simulink model "lv_demo7"  (Simulink 7.1)
settings: Solver=ode45  StartTime=0.0  StopTime=100  RelTol=1e-3
values from neighbouring files (symbols this model uses):
  C1 = 0.44    [lv_demofile.m]    (also in lv_demofile1.m; lv_demofile2.m; lv_demofile4.m; lv_demofile5.m)
  C2 = 0.0167    [lv_demofile.m]    (also in lv_demofile1.m; lv_demofile2.m; lv_demofile4.m; lv_demofile5.m)
  C3 = 0.3    [lv_demofile.m]    (also in lv_demofile1.m; lv_demofile2.m; lv_demofile4.m; lv_demofile5.m)
  C4 = 0.00184    [lv_demofile.m]    (also in lv_demofile1.m; lv_demofile2.m; lv_demofile4.m; lv_demofile5.m)
  Jem = 90    [lv_cankaofile.m]    (also in lv_demofile.m = 97.5; lv_demofile1.m = 97.5; lv_demofile2.m = 97.5; lv_demofile3.m = 97.5)
  Jwt = 9e7    (= 90000000)    [lv_cankaofile.m]    (also in lv_demofile.m = 3275300; lv_demofile1.m = 3275300; lv_demofile2.m = 3275300; lv_demofile3.m = 3275300)
  K = 83    [lv_cankaofile.m]    (also in lv_demofile.m; lv_demofile1.m = 75.76; lv_demofile2.m; lv_demofile3.m = 75.76)
  R = 40    [lv_cankaofile.m]    (also in lv_demofile.m = 38.5; lv_demofile1.m = 38.75; lv_demofile2.m = 38.5; lv_demofile3.m = 38.5)
  ro_air = 1.225    [lv_cankaofile.m]    (also in lv_demofile.m = 1.2236; lv_demofile1.m; lv_demofile2.m = 1.2236; lv_demofile3.m)
libraries: wt_blockset_v3 x2, simulink x1
settings Model: Creator=lv  LastModifiedBy=lv

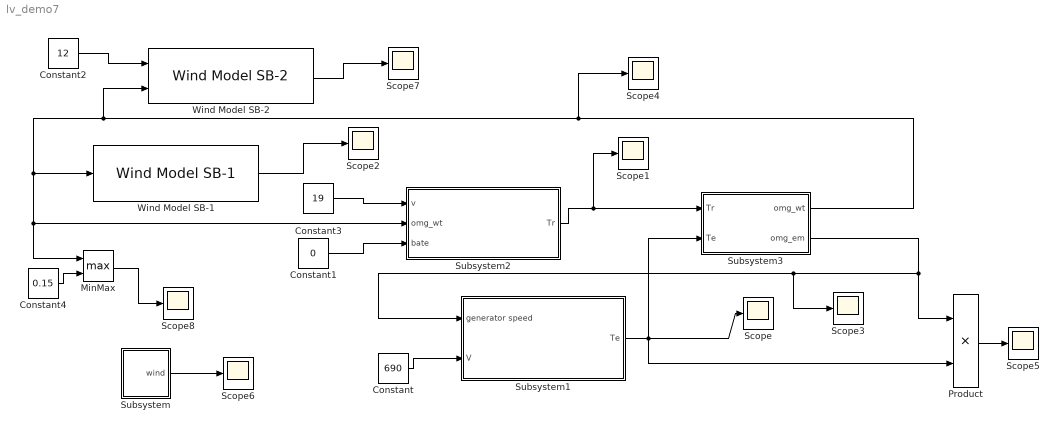
== system lv_demo7 ==
  Constant : Constant  Value=690  OutDataType=sfix(16)  OutScaling=2^0
  Constant1 : Constant  Value=0  OutDataType=sfix(16)  OutScaling=2^0
  Constant2 : Constant  Value=12  OutDataType=sfix(16)  OutScaling=2^0
  Constant3 : Constant  Value=19  OutDataType=sfix(16)  OutScaling=2^0
  Constant4 : Constant  Value=0.15  OutDataType=sfix(16)  OutScaling=2^0
  MinMax : MinMax  Function=max  Inputs=2  OutDataType=sfix(16)  OutScaling=2^0
  Product : Product  OutDataType=sfix(16)  OutScaling=2^0  RndMeth=Zero
  Scope{,1..8} (9 alike) : Scope
      Scope settings: YMin=0  YMax=100000
      Scope1 settings: TimeRange=12  YMin=-1.56503e+006  YMax=-1.56503e+006  SaveName=ScopeData2
      Scope2 settings: YMin=9.5  YMax=15  SaveName=ScopeData3
      Scope3 settings: SaveName=ScopeData5
      Scope4 settings: YMin=4.6  YMax=5.7  SaveName=ScopeData16
      Scope5 settings: TimeRange=100  YMin=-1.61921e+006  YMax=-1.61921e+006  SaveName=ScopeData9
      Scope6 settings: SaveName=ScopeData17
      Scope7 settings: SaveName=ScopeData18
      Scope8 settings: YMin=0.15  YMax=0.15  SaveName=ScopeData19
  Subsystem : Subsystem
  Subsystem1 : Subsystem
  Subsystem2 : Subsystem
  Subsystem3 : Subsystem
  Wind Model SB-1 : wt_blockset_v3/Mechanical Components/Wind Model SB-1  SystemSampleTime=-1  D_rotor=77  v_mean=13  roughness=600  turb_int=12  T_sample=0.01
  Wind Model SB-2 : wt_blockset_v3/Mechanical Components/Wind Model SB-2  SystemSampleTime=-1  D_rotor=77  L=600  turb_int=12  T_sample=0.05
  wires:
  Subsystem2/1(Tr) -> Scope1/1, Subsystem3/1(Tr)
  Subsystem3/2(omg_em) -> Product/1, Scope3/1, Subsystem1/1(generator speed)
  Subsystem1/1(Te) -> Scope/1, Subsystem3/2(Te), Product/2
  Subsystem3/1(omg_wt) -> Scope4/1, Wind Model SB-2/2, Wind Model SB-1/1, MinMax/1, Subsystem2/2(omg_wt)
  Constant/1 -> Subsystem1/2(V)
  Product/1 -> Scope5/1
  Constant1/1 -> Subsystem2/3(bate)
  Subsystem/1(wind) -> Scope6/1
  Constant2/1 -> Wind Model SB-2/1
  Wind Model SB-2/1 -> Scope7/1
  Wind Model SB-1/1 -> Scope2/1
  Constant4/1 -> MinMax/2
  MinMax/1 -> Scope8/1
  Constant3/1 -> Subsystem2/1(v)

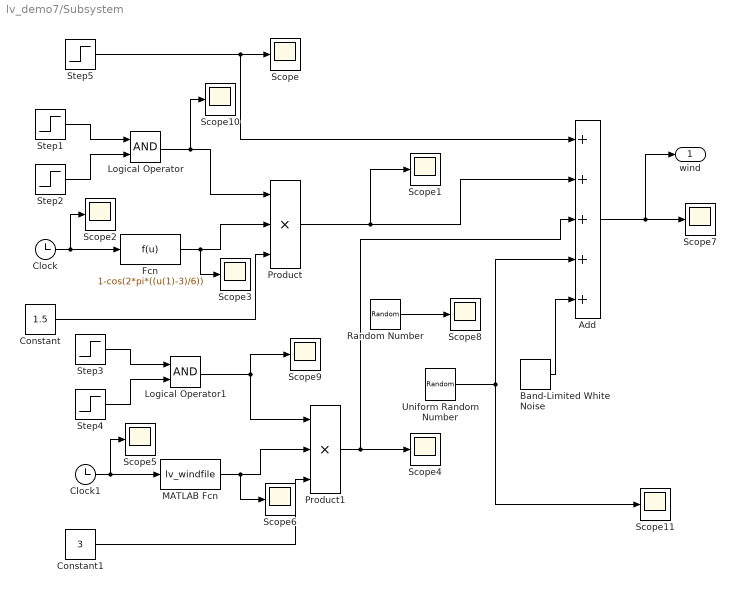
== system lv_demo7/Subsystem ==
  Add : Sum  Inputs=+++++  OutDataType=sfix(16)  OutScaling=2^-10
  Band-Limited White Noise : simulink/Sources/Band-Limited White Noise  SystemSampleTime=-1  Cov=[0.1]  Ts=0.1  seed=[23341]
  Clock : Clock
  Clock1 : Clock
  Constant : Constant  Value=1.5  OutDataType=sfix(16)  OutScaling=2^0
  Constant1 : Constant  Value=3  OutDataType=sfix(16)  OutScaling=2^0
  Fcn : Fcn  Expr=1-cos(2*pi*((u(1)-3)/6))
  Logical Operator : Logic  AllPortsSameDT=off  OutDataTypeMode=boolean  OutDataTypeStr=boolean
  Logical Operator1 : Logic  AllPortsSameDT=off  OutDataTypeMode=boolean  OutDataTypeStr=boolean
  MATLAB Fcn : MATLABFcn  MATLABFcn=lv_windfile
  Product : Product  Inputs=3  OutDataType=sfix(16)  OutScaling=2^0  RndMeth=Zero
  Product1 : Product  Inputs=3  OutDataType=sfix(16)  OutScaling=2^0  RndMeth=Zero
  Random Number : RandomNumber  Mean=5  SampleTime=0
  Scope{,1..11} (12 alike) : Scope
      Scope10 settings: SaveName=ScopeData11
      Scope11 settings: SaveName=ScopeData12
      Scope2 settings: SaveName=ScopeData2
      Scope3 settings: SaveName=ScopeData3
      Scope4 settings: SaveName=ScopeData4
      Scope5 settings: SaveName=ScopeData5
      Scope6 settings: SaveName=ScopeData6
      Scope7 settings: YMin=14.5  YMax=20  SaveName=ScopeData7
      Scope8 settings: SaveName=ScopeData8
      Scope9 settings: SaveName=ScopeData10
  Step1 : Step  Time=9  Before=1  After=0  SampleTime=0
  Step2 : Step  Time=3  SampleTime=0
  Step3 : Step  Time=11  Before=1  After=0  SampleTime=0
  Step4 : Step  Time=4  SampleTime=0
  Step5 : Step  Time=0  After=6  SampleTime=0
  Uniform Random Number : UniformRandomNumber  Minimum=7  Maximum=7.5  SampleTime=0
  wind : Outport  OutDataType=sfix(16)  OutScaling=2^0
  wires:
  Step5/1 -> Scope/1, Add/1
  Step1/1 -> Logical Operator/1
  Step2/1 -> Logical Operator/2
  Logical Operator/1 -> Product/1, Scope10/1
  Clock/1 -> Fcn/1, Scope2/1
  Fcn/1 -> Product/2, Scope3/1
  Constant/1 -> Product/3
  Product/1 -> Scope1/1, Add/2
  Step3/1 -> Logical Operator1/1
  Step4/1 -> Logical Operator1/2
  Logical Operator1/1 -> Product1/1, Scope9/1
  Clock1/1 -> Scope5/1, MATLAB Fcn/1
  MATLAB Fcn/1 -> Product1/2, Scope6/1
  Constant1/1 -> Product1/3
  Product1/1 -> Scope4/1, Add/3
  Add/1 -> Scope7/1, wind/1
  Random Number/1 -> Scope8/1
  Uniform Random Number/1 -> Scope11/1, Add/4
  Band-Limited White Noise/1 -> Add/5

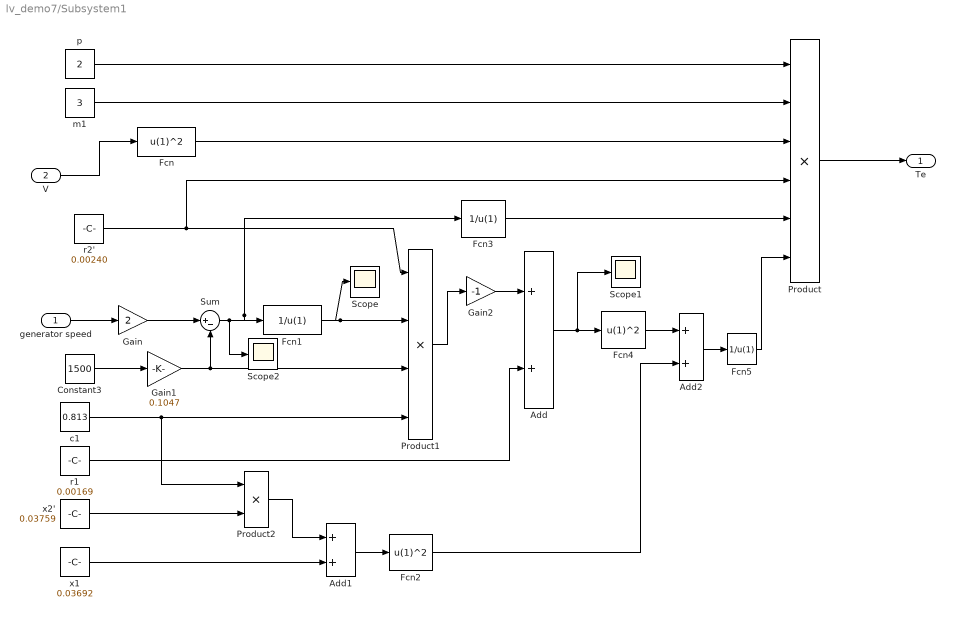
== system lv_demo7/Subsystem1 ==
  generator speed : Inport  OutDataType=sfix(16)  OutScaling=2^0
  V : Inport  Port=2  OutDataType=sfix(16)  OutScaling=2^0
  Add : Sum  OutDataType=sfix(16)  OutScaling=2^-10
  Add1 : Sum  OutDataType=sfix(16)  OutScaling=2^-10
  Add2 : Sum  OutDataType=sfix(16)  OutScaling=2^-10
  Constant3 : Constant  Value=1500  OutDataType=sfix(16)  OutScaling=2^0
  Fcn : Fcn  Expr=u(1)^2
  Fcn1 : Fcn  Expr=1/u(1)
  Fcn2 : Fcn  Expr=u(1)^2
  Fcn3 : Fcn  Expr=1/u(1)
  Fcn4 : Fcn  Expr=u(1)^2
  Fcn5 : Fcn  Expr=1/u(1)
  Gain : Gain  Gain=2  ParameterDataType=sfix(16)  ParameterScaling=2^0  OutDataType=sfix(16)  OutScaling=2^0
  Gain1 : Gain  Gain=0.1047  ParameterDataType=sfix(16)  ParameterScaling=2^0  OutDataType=sfix(16)  OutScaling=2^0
  Gain2 : Gain  Gain=-1  ParameterDataType=sfix(16)  ParameterScaling=2^0  OutDataType=sfix(16)  OutScaling=2^0
  Product : Product  Inputs=6  OutDataType=sfix(16)  OutScaling=2^0  RndMeth=Zero
  Product1 : Product  Inputs=4  OutDataType=sfix(16)  OutScaling=2^0  RndMeth=Zero
  Product2 : Product  OutDataType=sfix(16)  OutScaling=2^0  RndMeth=Zero
  Scope : Scope
      settings: YMin=0  YMax=100000  SaveName=ScopeData10
  Scope1 : Scope
      settings: YMin=0  YMax=100000  SaveName=ScopeData11
  Scope2 : Scope
      settings: YMin=0  YMax=100000  SaveName=ScopeData15
  Sum : Sum  Inputs=|+-  OutDataType=sfix(16)  OutScaling=2^0
  c1 : Constant  Value=0.813  OutDataType=sfix(16)  OutScaling=2^0
  m1 : Constant  Value=3  OutDataType=sfix(16)  OutScaling=2^0
  p : Constant  Value=2  OutDataType=sfix(16)  OutScaling=2^0
  r1 : Constant  Value=0.00169  OutDataType=sfix(16)  OutScaling=2^0
  r2' : Constant  Value=0.00240  OutDataType=sfix(16)  OutScaling=2^0
  x1 : Constant  Value=0.03692  OutDataType=sfix(16)  OutScaling=2^0
  x2' : Constant  Value=0.03759  OutDataType=sfix(16)  OutScaling=2^0
  Te : Outport  OutDataType=sfix(16)  OutScaling=2^0
  wires:
  V/1 -> Fcn/1
  generator speed/1 -> Gain/1
  Gain/1 -> Sum/1
  Constant3/1 -> Gain1/1
  Gain1/1 -> Sum/2, Product1/3
  Sum/1 -> Fcn3/1, Fcn1/1, Scope2/1
  r2'/1 -> Product1/1, Product/4
  c1/1 -> Product1/4, Product2/1
  x2'/1 -> Product2/2
  Product2/1 -> Add1/1
  x1/1 -> Add1/2
  Add1/1 -> Fcn2/1
  Product1/1 -> Gain2/1
  p/1 -> Product/1
  m1/1 -> Product/2
  Fcn/1 -> Product/3
  r1/1 -> Add/2
  Gain2/1 -> Add/1
  Fcn3/1 -> Product/5
  Add/1 -> Fcn4/1, Scope1/1
  Fcn4/1 -> Add2/1
  Fcn2/1 -> Add2/2
  Add2/1 -> Fcn5/1
  Fcn5/1 -> Product/6
  Product/1 -> Te/1
  Fcn1/1 -> Product1/2, Scope/1

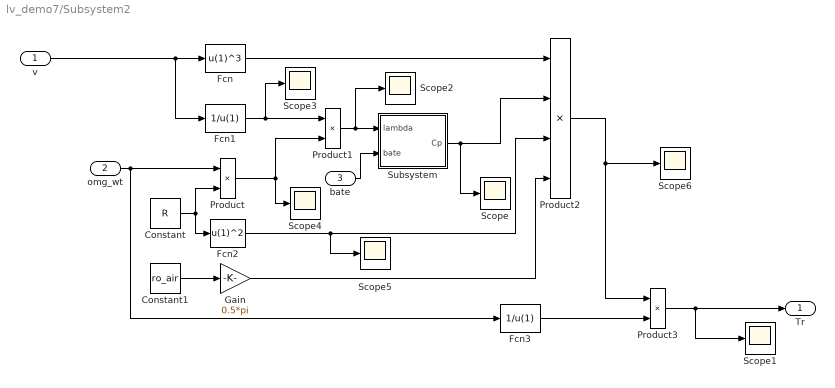
== system lv_demo7/Subsystem2 ==
  v : Inport  OutDataType=sfix(16)  OutScaling=2^0
  omg_wt : Inport  Port=2  OutDataType=sfix(16)  OutScaling=2^0
  bate : Inport  Port=3  OutDataType=sfix(16)  OutScaling=2^0
  Constant : Constant  Value=R  OutDataType=sfix(16)  OutScaling=2^0
  Constant1 : Constant  Value=ro_air  OutDataType=sfix(16)  OutScaling=2^0
  Fcn : Fcn  Expr=u(1)^3
  Fcn1 : Fcn  Expr=1/u(1)
  Fcn2 : Fcn  Expr=u(1)^2
  Fcn3 : Fcn  Expr=1/u(1)
  Gain : Gain  Gain=0.5*pi  ParameterDataType=sfix(16)  ParameterScaling=2^0  OutDataType=sfix(16)  OutScaling=2^0
  Product : Product  OutDataType=sfix(16)  OutScaling=2^0  RndMeth=Zero
  Product1 : Product  OutDataType=sfix(16)  OutScaling=2^0  RndMeth=Zero
  Product2 : Product  Inputs=4  OutDataType=sfix(16)  OutScaling=2^0  RndMeth=Zero
  Product3 : Product  OutDataType=sfix(16)  OutScaling=2^0  RndMeth=Zero
  Scope{,1..6} (7 alike) : Scope
      Scope settings: TimeRange=50  YMin=0.1772981595092024  YMax=0.2028981595092024  SaveName=ScopeData4
      Scope1 settings: TimeRange=20  YMin=-1500000  YMax=1500000
      Scope2 settings: SaveName=ScopeData6
      Scope3 settings: SaveName=ScopeData7
      Scope4 settings: SaveName=ScopeData8
      Scope5 settings: YMin=1501.56  YMax=1501.56  SaveName=ScopeData20
      Scope6 settings: TimeRange=20  YMin=-500000  YMax=5e+006  SaveName=ScopeData21
  Subsystem : Subsystem
  Tr : Outport  OutDataType=sfix(16)  OutScaling=2^0
  wires:
  v/1 -> Fcn/1, Fcn1/1
  omg_wt/1 -> Product/1, Fcn3/1
  Constant/1 -> Product/2, Fcn2/1
  Fcn1/1 -> Product1/1, Scope3/1
  Product/1 -> Product1/2, Scope4/1
  Product1/1 -> Subsystem/1(lambda), Scope2/1
  bate/1 -> Subsystem/2(bate)
  Fcn/1 -> Product2/1
  Subsystem/1(Cp) -> Product2/2, Scope/1
  Fcn2/1 -> Product2/3, Scope5/1
  Gain/1 -> Product2/4
  Constant1/1 -> Gain/1
  Product2/1 -> Product3/1, Scope6/1
  Fcn3/1 -> Product3/2
  Product3/1 -> Scope1/1, Tr/1

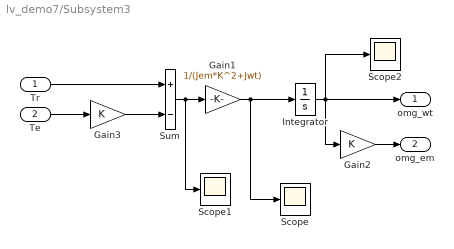
== system lv_demo7/Subsystem3 ==
  Tr : Inport  OutDataType=sfix(16)  OutScaling=2^0
  Te : Inport  Port=2  OutDataType=sfix(16)  OutScaling=2^0
  Gain1 : Gain  Gain=1/(Jem*K^2+Jwt)  ParameterDataType=sfix(16)  ParameterScaling=2^0  OutDataType=sfix(16)  OutScaling=2^0  SaturateOnIntegerOverflow=on  OutDataTypeStr=Inherit: Same as input  ParamDataTypeStr=Inherit: Same as input
  Gain2 : Gain  Gain=K  ParameterDataType=sfix(16)  ParameterScaling=2^0  OutDataType=sfix(16)  OutScaling=2^0  SaturateOnIntegerOverflow=on  OutDataTypeStr=Inherit: Same as input  ParamDataTypeStr=Inherit: Same as input
  Gain3 : Gain  Gain=K  ParameterDataType=sfix(16)  ParameterScaling=2^0  OutDataType=sfix(16)  OutScaling=2^0  SaturateOnIntegerOverflow=on  OutDataTypeStr=Inherit: Same as input  ParamDataTypeStr=Inherit: Same as input
  Integrator : Integrator  InitialCondition=1  UpperSaturationLimit=0.95*2*pi*60  LowerSaturationLimit=0
  Scope : Scope
      settings: YMin=0  YMax=100000  SaveName=ScopeData12
  Scope1 : Scope
      settings: YMin=0  YMax=100000  SaveName=ScopeData13
  Scope2 : Scope
      settings: YMin=-0.025  YMax=0.035  SaveName=ScopeData14
  Sum : Sum  Inputs=+-  OutDataType=sfix(16)  OutScaling=2^0  SaturateOnIntegerOverflow=on  InputSameDT=on  OutDataTypeStr=Inherit: Same as first input
  omg_wt : Outport  OutDataType=sfix(16)  OutScaling=2^0  InitialOutput=0
  omg_em : Outport  Port=2  OutDataType=sfix(16)  OutScaling=2^0  InitialOutput=0
  wires:
  Gain1/1 -> Integrator/1, Scope/1
  Sum/1 -> Gain1/1, Scope1/1
  Te/1 -> Gain3/1
  Tr/1 -> Sum/1
  Gain2/1 -> omg_em/1
  Gain3/1 -> Sum/2
  Integrator/1 -> omg_wt/1, Gain2/1, Scope2/1

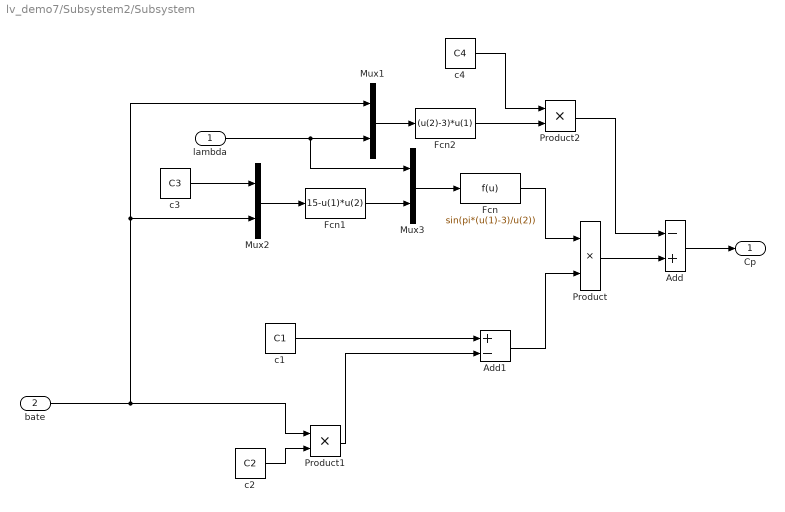
== system lv_demo7/Subsystem2/Subsystem ==
  lambda : Inport  OutDataType=sfix(16)  OutScaling=2^0
  bate : Inport  Port=2  OutDataType=sfix(16)  OutScaling=2^0
  Add : Sum  Inputs=-+  OutDataType=sfix(16)  OutScaling=2^-10
  Add1 : Sum  Inputs=+-  OutDataType=sfix(16)  OutScaling=2^-10
  Fcn : Fcn  Expr=sin(pi*(u(1)-3)/u(2))
  Fcn1 : Fcn  Expr=15-u(1)*u(2)
  Fcn2 : Fcn  Expr=(u(2)-3)*u(1)
  Mux1 : Mux  Inputs=2
  Mux2 : Mux  Inputs=2
  Mux3 : Mux  Inputs=2
  Product : Product  OutDataType=sfix(16)  OutScaling=2^0  RndMeth=Zero
  Product1 : Product  OutDataType=sfix(16)  OutScaling=2^0  RndMeth=Zero
  Product2 : Product  OutDataType=sfix(16)  OutScaling=2^0  RndMeth=Zero
  c1 : Constant  Value=C1  OutDataType=sfix(16)  OutScaling=2^0
  c2 : Constant  Value=C2  OutDataType=sfix(16)  OutScaling=2^0
  c3 : Constant  Value=C3  OutDataType=sfix(16)  OutScaling=2^0
  c4 : Constant  Value=C4  OutDataType=sfix(16)  OutScaling=2^0
  Cp : Outport  OutDataType=sfix(16)  OutScaling=2^0
  wires:
  Add/1 -> Cp/1
  Product2/1 -> Add/1
  Fcn2/1 -> Product2/2
  c4/1 -> Product2/1
  Mux1/1 -> Fcn2/1
  lambda/1 -> Mux1/2, Mux3/1
  Fcn1/1 -> Mux3/2
  Product/1 -> Add/2
  Add1/1 -> Product/2
  Fcn/1 -> Product/1
  Mux3/1 -> Fcn/1
  c3/1 -> Mux2/1
  Mux2/1 -> Fcn1/1
  Product1/1 -> Add1/2
  c2/1 -> Product1/2
  bate/1 -> Mux1/1, Mux2/2, Product1/1
  c1/1 -> Add1/1
